simulink model "ControllerExample"  (R2019b)
settings: Solver=VariableStepAuto  StartTime=0.0  StopTime=10.0  RelTol=1e-3
undefined symbols (not defined in the file): Ki, Kx
settings Model: Creator=Sankalp Bhan  LastModifiedBy=Sankalp Bhan

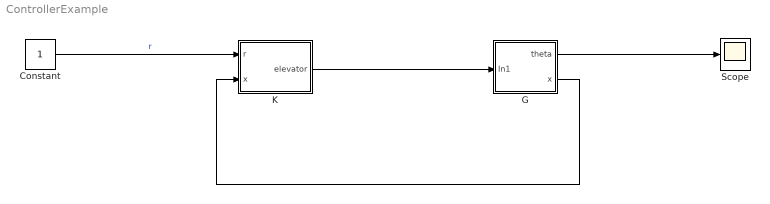
== system ControllerExample ==
  Constant : Constant
  G : Subsystem
  K : Subsystem
  Scope : Scope
  wires:
  Constant/1 -> K/1(r)  "r"
  K/1(elevator) -> G/1(In1)
  G/1(theta) -> Scope/1
  G/2(x) -> K/2(x)

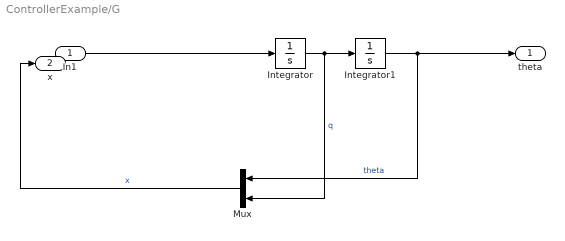
== system ControllerExample/G ==
  In1 : Inport
  Integrator : Integrator
  Integrator1 : Integrator
  Mux : Mux  Inputs=2
  theta : Outport
  x : Outport  Port=2
  wires:
  Integrator/1 -> Mux/2, Integrator1/1  "q"
  In1/1 -> Integrator/1
  Integrator1/1 -> theta/1, Mux/1  "theta"
  Mux/1 -> x/1  "x"

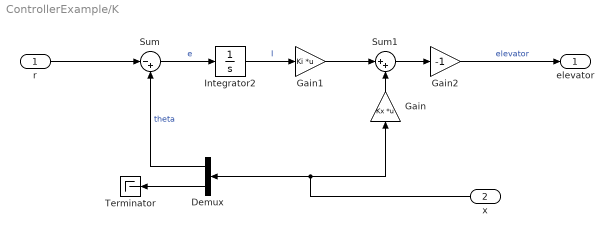
== system ControllerExample/K ==
  r : Inport
  x : Inport  Port=2
  Demux : Demux  Outputs=2
  Gain : Gain  Gain=Kx  Multiplication=Matrix(K*u)
  Gain1 : Gain  Gain=Ki  Multiplication=Matrix(K*u)
  Gain2 : Gain  Gain=-1
  Integrator2 : Integrator
  Sum : Sum  Inputs=|-+
  Sum1 : Sum  Inputs=|++
  Terminator : Terminator
  elevator : Outport
  wires:
  r/1 -> Sum/1
  Sum1/1 -> Gain2/1
  x/1 -> Demux/1, Gain/1
  Integrator2/1 -> Gain1/1  "I"
  Gain1/1 -> Sum1/1
  Demux/2 -> Terminator/1
  Gain/1 -> Sum1/2
  Sum/1 -> Integrator2/1  "e"
  Demux/1 -> Sum/2  "theta"
  Gain2/1 -> elevator/1  "elevator"
